simulink library "SMC"  (R2017b)
settings: Solver=VariableStepAuto  StartTime=0.0  StopTime=10.0  RelTol=1e-3
undefined symbols (not defined in the file or in its folder): A, B, beta, C, C0, filter, gamma0, K0, k02, K1, K2, K3, p, P2, PC, Pk, pk, rho, S, Slat, yc
libraries: dspmtrx3 x18
settings Model: Creator=lev201  LastModifiedBy=Liam Uni

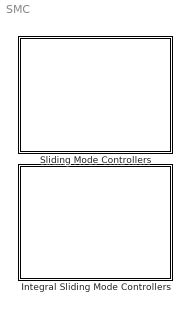
== system SMC ==
  Integral Sliding Mode Controllers : Subsystem
      mask Display: disp('Integral Sliding Mode Controllers')
  Sliding Mode Controllers : Subsystem
      mask Display: disp('Sliding Mode Controllers')

== system SMC/Integral Sliding Mode Controllers ==
  AISMC : Subsystem  mask{A=A, B=B, C=C, S=S, rho=rho, P2=P2, delta=0, eps=0, c0=C0, k0=K0, pc=PC, pk=Pk, filter=filter, yc=0}
      mask prompts: A "System Matrix (A)"; B "Effectiveness Matrix (B)"; C "Output Matrix (C)"; S "Sliding Surface (S)"; pc "Learning rate of c estimate"; pk "Learning rate of k estimation"
      mask init:
      | [K1 K2 K3]=SMCgains(S, A, B, C, yc, P2)
      mask DialogControl DescGroupVar Prompt: Adaptive Integral Sliding Mode Controller
      mask DialogControl DescTextVar Prompt: This controller gaurantees sliding as long as: rho>=||uncertainty|| A sigmoidal function can be used to create a continuous pseudo-sliding non-linear component using delta: sig(s)=P2s/(||P2s||+delta). A boundary layer around the sliding surface can be used using eps: if ||P2s||>eps un(t)=un(t) if ||P2s||<=eps, un(t)=0. An adaptive method is used to estimate the bounds of matched uncertaintym such that ||fm(x,u,t)||<=C1+K1||x(t)||. Integral action is introduced for the outputs yc.
      mask DialogControl Container4 Prompt: Model Parameters
      mask DialogControl Container6 Prompt: Controller Parameters
      mask DialogControl Container11 Prompt: Gain Tuning
      mask DialogControl Container12 Prompt: Chattering Avoidance
      mask DialogControl Container14 Prompt: Adaptive Parmeters
      mask DialogControl Container15 Prompt: Reference Tracking
      mask Display:
      | disp('AISMC')
      | port_label('input', 1, 'x(t)');
      | port_label('output', 1, 'u(t)');
      | port_label('output', 2, 's(t)');
      | port_label('output', 3, 'AP');
      | port_label('input', 2, 'R(t)');
  ISMC : Subsystem  mask{A=A, B=B, C=C, S=S, rho=rho, P2=P2, delta=0, eps=0, filter=filter, yc=yc}
      mask prompts: A "System Matrix (A)"; B "Effectiveness Matrix (B)"; C "Output Matrix (C)"; S "Sliding Surface (S)"
      mask init:
      | [K1 K2 K3]=SMCgains(S, A, B, C, yc, P2)
      mask DialogControl DescGroupVar Prompt: Integral Sliding Mode Controller
      mask DialogControl DescTextVar Prompt: This controller gaurantees sliding as long as: rho>=||uncertainty|| A sigmoidal function can be used to create a continuous pseudo-sliding non-linear component using delta: sig(s)=P2s/(||P2s||+delta).  A boundary layer around the sliding surface can be used using eps: if ||P2s||>eps un(t)=un(t) if ||P2s||<=eps un(t)=0. Integral action is introduced for the outputs yc.
      mask DialogControl Container4 Prompt: Model Parameters
      mask DialogControl Container6 Prompt: Controller Parameters
      mask DialogControl Container11 Prompt: Gain Tuning
      mask DialogControl Container12 Prompt: Chattering Avoidance
      mask DialogControl Container13 Prompt: Reference Tracking
      mask Display:
      | disp('ISMC')
      | port_label('input', 1, 'x(t)');
      | port_label('input', 2, 'R(t)');
      | 
      | port_label('output', 1, 'u(t)');
      | port_label('output', 2, 's(t)');
  SRAISMC : Subsystem  mask{A=A, B=B, C=C, S=S, rho=rho, P2=P2, delta=0, eps=0, c0=C0, gamma0=gamma0, pc=PC, beta=beta, filter=filter, yc=yc}
      mask prompts: A "System Matrix (A)"; B "Effectiveness Matrix (B)"; C "Output  Matrix (C)"; S "Sliding Surface (S)"; pc "Learning rate of c estimate"; beta "Adaptive rate"
      mask init:
      | [K1 K2 K3]=SMCgains(S, A, B, C, yc, P2)
      mask DialogControl DescGroupVar Prompt: Saturation Robust Adaptive Integral Sliding Mode Controller
      mask DialogControl DescTextVar Prompt: This controller gaurantees sliding as long as: rho>=||uncertainty|| A sigmoidal function can be used to create a continuous pseudo-sliding non-linear component using delta: sig(s)=P2s/(||P2s||+delta). A boundary layer around the sliding surface can be used using eps: if ||P2s||>eps un(t)=un(t) if ||P2s||<=eps, un(t)=0. An adaptive method is used to estimate the bounds of matched uncertaintym such that ||fm(x,u,t)||<=C1+K1||x(t)||.
      mask DialogControl Container4 Prompt: Model Parameters
      mask DialogControl Container6 Prompt: Controller Parameters
      mask DialogControl Container11 Prompt: Gain Tuning
      mask DialogControl Container12 Prompt: Chattering Avoidance
      mask DialogControl Container14 Prompt: Adaptive Parmeters
      mask DialogControl Container15 Prompt: Reference Tracking
      mask Display:
      | disp('SRAISMC')
      | port_label('input', 1, 'x(t)');
      | port_label('output', 1, 'u(t)');
      | port_label('output', 2, 's(t)');
      | port_label('output', 3, 'AP');
      | port_label('input', 2, 'R(t)');

== system SMC/Sliding Mode Controllers ==
  ASMC : Subsystem  mask{A=A, B=B, S=S, rho=rho, P2=P2, delta=0, eps=0, c0=C0, k0=K0, pc=PC, pk=Pk}
      mask prompts: A "System Matrix (A)"; B "Effectiveness Matrix (B)"; S "Sliding Surface (S)"; pc "Learning rate of c estimate"; pk "Learning rate of k estimation"
      mask init:
      | [K1 K2]=SMCgains(S, A, B, P2)
      mask DialogControl DescGroupVar Prompt: Adaptive Sliding Mode Controller
      mask DialogControl DescTextVar Prompt: This controller gaurantees sliding as long as: rho>=||uncertainty|| A sigmoidal function can be used to create a continuous pseudo-sliding non-linear component using delta: sig(s)=P2s/(||P2s||+delta). A boundary layer around the sliding surface can be used using eps: if ||P2s||>eps un(t)=un(t) if ||P2s||<=eps, un(t)=0. An adaptive method is used to estimate the bounds of matched uncertaintym such that ||fm(x,u,t)||<=C1+K1||x(t)||.
      mask DialogControl Container4 Prompt: Model Parameters
      mask DialogControl Container6 Prompt: Controller Parameters
      mask DialogControl Container11 Prompt: Gain Tuning
      mask DialogControl Container12 Prompt: Chattering Avoidance
      mask DialogControl Container14 Prompt: Adaptive Parmeters
      mask Display:
      | disp('ASMC')
      | port_label('input', 1, 'x(t)');
      | port_label('output', 1, 'u(t)');
      | port_label('output', 2, 's(t)');
      | port_label('output', 3, 'AP');
  SMC : Subsystem  mask{A=A, B=B, S=S, rho=rho, P2=P2, delta=0, eps=0}
      mask prompts: A "System Matrix (A)"; B "Effectiveness Matrix (B)"; S "Sliding Surface (S)"
      mask init:
      | [K1 K2]=SMCgains(S, A, B, P2)
      mask DialogControl DescGroupVar Prompt: Sliding Mode Controller
      mask DialogControl DescTextVar Prompt: This controller gaurantees sliding as long as: rho>=||uncertainty|| A sigmoidal function can be used to create a continuous pseudo-sliding non-linear component using delta: sig(s)=P2s/(||P2s||+delta).  A boundary layer around the sliding surface can be used using eps: if ||P2s||>eps un(t)=un(t) if ||P2s||<=eps un(t)=0
      mask DialogControl Container4 Prompt: Model Parameters
      mask DialogControl Container6 Prompt: Controller Parameters
      mask DialogControl Container11 Prompt: Gain Tuning
      mask DialogControl Container12 Prompt: Chattering Avoidance
      mask Display:
      | disp('SMC')
      | port_label('input', 1, 'x(t)');
      | port_label('output', 1, 'u(t)');
      | port_label('output', 2, 's(t)');
  SRASMC : Subsystem  mask{A=A, B=B, S=S, rho=rho, P2=P2, delta=0, eps=0, c0=C0, gamma0=gamma0, pc=PC, beta=beta}
      mask prompts: A "System Matrix (A)"; B "Effectiveness Matrix (B)"; S "Sliding Surface (S)"; pc "Learning rate of c estimate"; beta "Adaptive rate"
      mask init:
      | [K1 K2]=SMCgains(S, A, B, P2)
      mask DialogControl DescGroupVar Prompt: Saturation Robust Adaptive Sliding Mode Controller
      mask DialogControl DescTextVar Prompt: This controller gaurantees sliding as long as: rho>=||uncertainty|| A sigmoidal function can be used to create a continuous pseudo-sliding non-linear component using delta: sig(s)=P2s/(||P2s||+delta). A boundary layer around the sliding surface can be used using eps: if ||P2s||>eps un(t)=un(t) if ||P2s||<=eps, un(t)=0. An adaptive method is used to estimate the bounds of matched uncertaintym such that ||fm(x,u,t)||<=C1+K1||x(t)||.
      mask DialogControl Container4 Prompt: Model Parameters
      mask DialogControl Container6 Prompt: Controller Parameters
      mask DialogControl Container11 Prompt: Gain Tuning
      mask DialogControl Container12 Prompt: Chattering Avoidance
      mask DialogControl Container14 Prompt: Adaptive Parmeters
      mask Display:
      | disp('SRASMC')
      | port_label('input', 1, 'x(t)');
      | port_label('output', 1, 'u(t)');
      | port_label('output', 2, 's(t)');
      | port_label('output', 3, 'AP');

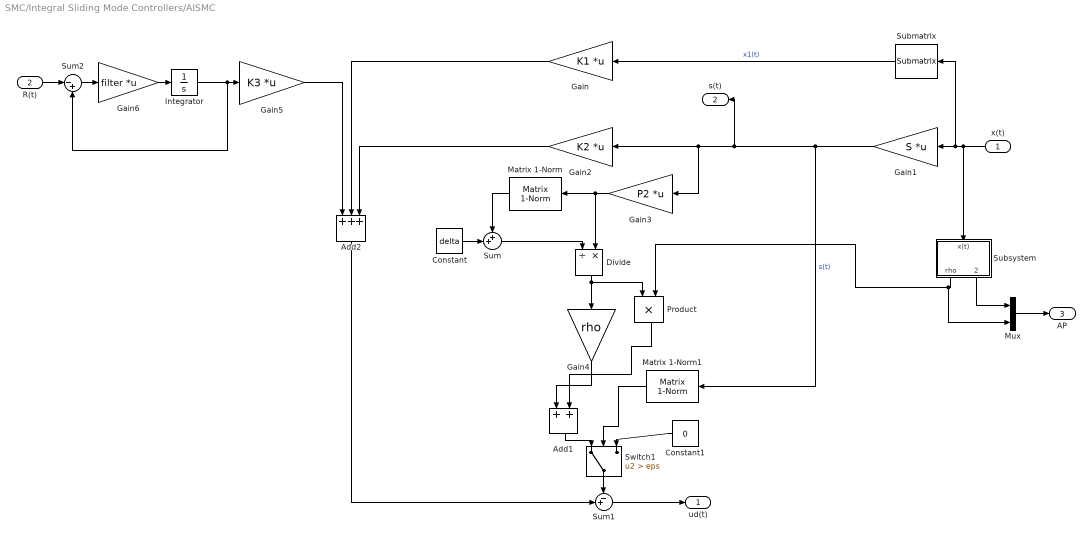
== system SMC/Integral Sliding Mode Controllers/AISMC ==
  x(t) : Inport
  R(t) : Inport  Port=2
  Add1 : Sum
  Add2 : Sum  Inputs=+++
  Constant : Constant  Value=delta
  Constant1 : Constant  Value=0
  Divide : Product  Inputs=/*
  Gain : Gain  Gain=K1  Multiplication=Matrix(K*u) (u vector)
  Gain1 : Gain  Gain=S  Multiplication=Matrix(K*u) (u vector)
  Gain2 : Gain  Gain=K2  Multiplication=Matrix(K*u) (u vector)
  Gain3 : Gain  Gain=P2  Multiplication=Matrix(K*u) (u vector)
  Gain4 : Gain  Gain=rho
  Gain5 : Gain  Gain=K3  Multiplication=Matrix(K*u) (u vector)
  Gain6 : Gain  Gain=filter  Multiplication=Matrix(K*u) (u vector)
  Integrator : Integrator
  Matrix 1-Norm : dspmtrx3/Matrix  1-Norm  outputDataTypeStr=Inherit: Same as accumulator  outputLastDataTypeStr=Inherit: Same as accumulator  outputMin=[]  outputMax=[]  roundingMode=Floor  overflowMode=off
      settings: SourceProductName=DSP System Toolbox  SourceProductBaseCode=DS
  Matrix 1-Norm1 : dspmtrx3/Matrix  1-Norm  outputDataTypeStr=Inherit: Same as accumulator  outputLastDataTypeStr=Inherit: Same as accumulator  outputMin=[]  outputMax=[]  roundingMode=Floor  overflowMode=off
      settings: SourceProductName=DSP System Toolbox  SourceProductBaseCode=DS
  Mux : Mux  Inputs=2
  Product : Product
  Submatrix : dspmtrx3/Submatrix  RowSpan=Range of rows  RowStartMode=Index  RowStartIndex=1  RowEndMode=Index  RowEndIndex=p-1  ColSpan=All columns  ColStartMode=First  ColStartIndex=1  ColEndMode=Last  ColEndIndex=1
  Subsystem : Subsystem
  Sum : Sum  Inputs=++|
  Sum1 : Sum  Inputs=-+|
  Sum2 : Sum  Inputs=|-+
  Switch1 : Switch  Criteria=u2 > Threshold  Threshold=eps  ZeroCross=off
  ud(t) : Outport
  s(t) : Outport  Port=2
  AP : Outport  Port=3
  wires:
  Gain1/1 -> Matrix 1-Norm1/1, Gain2/1, Gain3/1, s(t)/1  "s(t)"
  Divide/1 -> Product/1, Gain4/1
  Constant/1 -> Sum/2
  Matrix 1-Norm/1 -> Sum/1
  Gain4/1 -> Add1/1
  Sum/1 -> Divide/1
  Sum1/1 -> ud(t)/1
  Gain3/1 -> Matrix 1-Norm/1, Divide/2
  Switch1/1 -> Sum1/1
  Matrix 1-Norm1/1 -> Switch1/2
  Constant1/1 -> Switch1/3
  x(t)/1 -> Subsystem/1(x(t)), Submatrix/1, Gain1/1
  Submatrix/1 -> Gain/1  "x1(t)"
  Subsystem/1(rho) -> Mux/2, Product/2
  Add1/1 -> Switch1/1
  Product/1 -> Add1/2
  Subsystem/2(est-par) -> Mux/1
  Mux/1 -> AP/1
  Sum2/1 -> Gain6/1
  Gain5/1 -> Add2/1
  Gain6/1 -> Integrator/1
  Add2/1 -> Sum1/2
  Gain2/1 -> Add2/3
  Gain/1 -> Add2/2
  Integrator/1 -> Sum2/2, Gain5/1
  R(t)/1 -> Sum2/1

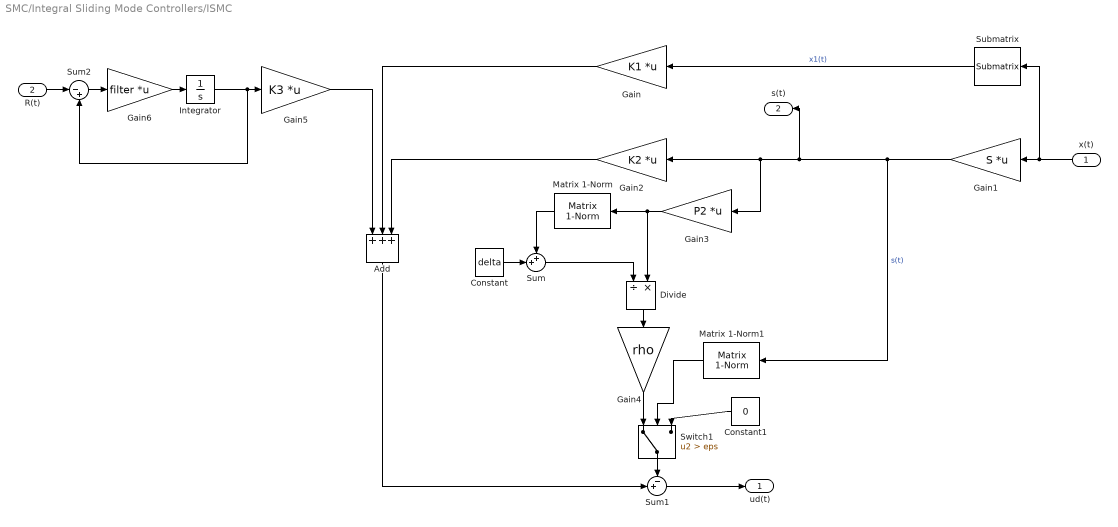
== system SMC/Integral Sliding Mode Controllers/ISMC ==
  x(t) : Inport
  R(t) : Inport  Port=2
  Add : Sum  Inputs=+++
  Constant : Constant  Value=delta
  Constant1 : Constant  Value=0
  Divide : Product  Inputs=/*
  Gain : Gain  Gain=K1  Multiplication=Matrix(K*u) (u vector)
  Gain1 : Gain  Gain=S  Multiplication=Matrix(K*u) (u vector)
  Gain2 : Gain  Gain=K2  Multiplication=Matrix(K*u) (u vector)
  Gain3 : Gain  Gain=P2  Multiplication=Matrix(K*u) (u vector)
  Gain4 : Gain  Gain=rho
  Gain5 : Gain  Gain=K3  Multiplication=Matrix(K*u) (u vector)
  Gain6 : Gain  Gain=filter  Multiplication=Matrix(K*u) (u vector)
  Integrator : Integrator
  Matrix 1-Norm : dspmtrx3/Matrix  1-Norm  outputDataTypeStr=Inherit: Same as accumulator  outputLastDataTypeStr=Inherit: Same as accumulator  outputMin=[]  outputMax=[]  roundingMode=Floor  overflowMode=off
      settings: SourceProductName=DSP System Toolbox  SourceProductBaseCode=DS
  Matrix 1-Norm1 : dspmtrx3/Matrix  1-Norm  outputDataTypeStr=Inherit: Same as accumulator  outputLastDataTypeStr=Inherit: Same as accumulator  outputMin=[]  outputMax=[]  roundingMode=Floor  overflowMode=off
      settings: SourceProductName=DSP System Toolbox  SourceProductBaseCode=DS
  Submatrix : dspmtrx3/Submatrix  RowSpan=Range of rows  RowStartMode=Index  RowStartIndex=1  RowEndMode=Index  RowEndIndex=p-1  ColSpan=All columns  ColStartMode=First  ColStartIndex=1  ColEndMode=Last  ColEndIndex=1
  Sum : Sum  Inputs=++|
  Sum1 : Sum  Inputs=-+|
  Sum2 : Sum  Inputs=|-+
  Switch1 : Switch  Criteria=u2 > Threshold  Threshold=eps  ZeroCross=off
  ud(t) : Outport
  s(t) : Outport  Port=2
  wires:
  Gain1/1 -> Matrix 1-Norm1/1, Gain2/1, Gain3/1, s(t)/1  "s(t)"
  Divide/1 -> Gain4/1
  Constant/1 -> Sum/2
  Matrix 1-Norm/1 -> Sum/1
  Add/1 -> Sum1/2
  Gain2/1 -> Add/3
  Gain4/1 -> Switch1/1
  Sum/1 -> Divide/1
  Sum1/1 -> ud(t)/1
  Gain3/1 -> Matrix 1-Norm/1, Divide/2
  Switch1/1 -> Sum1/1
  Matrix 1-Norm1/1 -> Switch1/2
  Constant1/1 -> Switch1/3
  x(t)/1 -> Submatrix/1, Gain1/1
  Submatrix/1 -> Gain/1  "x1(t)"
  Gain/1 -> Add/2
  Integrator/1 -> Sum2/2, Gain5/1
  Gain5/1 -> Add/1
  R(t)/1 -> Sum2/1
  Sum2/1 -> Gain6/1
  Gain6/1 -> Integrator/1

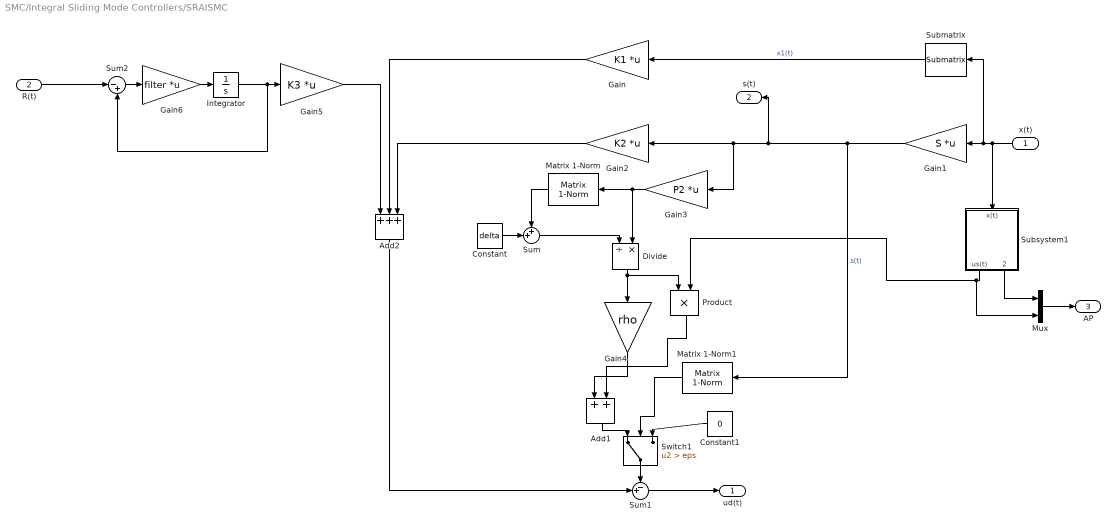
== system SMC/Integral Sliding Mode Controllers/SRAISMC ==
  x(t) : Inport
  R(t) : Inport  Port=2
  Add1 : Sum
  Add2 : Sum  Inputs=+++
  Constant : Constant  Value=delta
  Constant1 : Constant  Value=0
  Divide : Product  Inputs=/*
  Gain : Gain  Gain=K1  Multiplication=Matrix(K*u) (u vector)
  Gain1 : Gain  Gain=S  Multiplication=Matrix(K*u) (u vector)
  Gain2 : Gain  Gain=K2  Multiplication=Matrix(K*u) (u vector)
  Gain3 : Gain  Gain=P2  Multiplication=Matrix(K*u) (u vector)
  Gain4 : Gain  Gain=rho
  Gain5 : Gain  Gain=K3  Multiplication=Matrix(K*u) (u vector)
  Gain6 : Gain  Gain=filter  Multiplication=Matrix(K*u) (u vector)
  Integrator : Integrator
  Matrix 1-Norm : dspmtrx3/Matrix  1-Norm  outputDataTypeStr=Inherit: Same as accumulator  outputLastDataTypeStr=Inherit: Same as accumulator  outputMin=[]  outputMax=[]  roundingMode=Floor  overflowMode=off
      settings: SourceProductName=DSP System Toolbox  SourceProductBaseCode=DS
  Matrix 1-Norm1 : dspmtrx3/Matrix  1-Norm  outputDataTypeStr=Inherit: Same as accumulator  outputLastDataTypeStr=Inherit: Same as accumulator  outputMin=[]  outputMax=[]  roundingMode=Floor  overflowMode=off
      settings: SourceProductName=DSP System Toolbox  SourceProductBaseCode=DS
  Mux : Mux  Inputs=2
  Product : Product
  Submatrix : dspmtrx3/Submatrix  RowSpan=Range of rows  RowStartMode=Index  RowStartIndex=1  RowEndMode=Index  RowEndIndex=p-1  ColSpan=All columns  ColStartMode=First  ColStartIndex=1  ColEndMode=Last  ColEndIndex=1
  Subsystem1 : Subsystem
  Sum : Sum  Inputs=++|
  Sum1 : Sum  Inputs=-+|
  Sum2 : Sum  Inputs=|-+
  Switch1 : Switch  Criteria=u2 > Threshold  Threshold=eps  ZeroCross=off
  ud(t) : Outport
  s(t) : Outport  Port=2
  AP : Outport  Port=3
  wires:
  Mux/1 -> AP/1
  Subsystem1/2(est-par) -> Mux/1
  Product/1 -> Add1/2
  Add1/1 -> Switch1/1
  Subsystem1/1(us(t)) -> Product/2, Mux/2
  Gain/1 -> Add2/2
  Submatrix/1 -> Gain/1  "x1(t)"
  x(t)/1 -> Subsystem1/1(x(t)), Gain1/1, Submatrix/1
  Constant1/1 -> Switch1/3
  Matrix 1-Norm1/1 -> Switch1/2
  Switch1/1 -> Sum1/1
  Gain3/1 -> Divide/2, Matrix 1-Norm/1
  Sum1/1 -> ud(t)/1
  Sum/1 -> Divide/1
  Gain4/1 -> Add1/1
  Gain2/1 -> Add2/3
  Matrix 1-Norm/1 -> Sum/1
  Constant/1 -> Sum/2
  Divide/1 -> Gain4/1, Product/1
  Gain1/1 -> s(t)/1, Gain3/1, Gain2/1, Matrix 1-Norm1/1  "s(t)"
  Integrator/1 -> Sum2/2, Gain5/1
  R(t)/1 -> Sum2/1
  Gain6/1 -> Integrator/1
  Sum2/1 -> Gain6/1
  Gain5/1 -> Add2/1
  Add2/1 -> Sum1/2

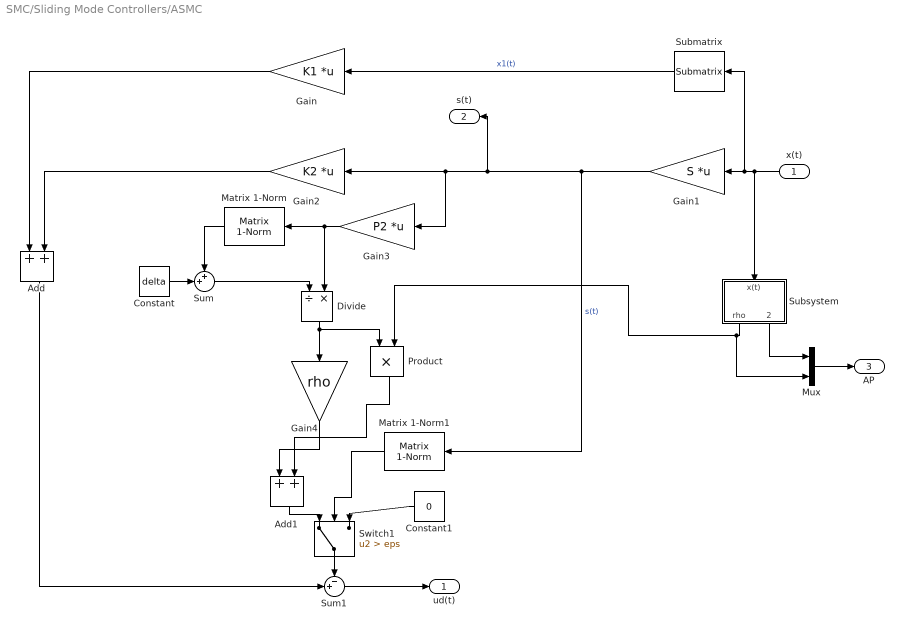
== system SMC/Sliding Mode Controllers/ASMC ==
  x(t) : Inport
  Add : Sum
  Add1 : Sum
  Constant : Constant  Value=delta
  Constant1 : Constant  Value=0
  Divide : Product  Inputs=/*
  Gain : Gain  Gain=K1  Multiplication=Matrix(K*u) (u vector)
  Gain1 : Gain  Gain=S  Multiplication=Matrix(K*u) (u vector)
  Gain2 : Gain  Gain=K2  Multiplication=Matrix(K*u) (u vector)
  Gain3 : Gain  Gain=P2  Multiplication=Matrix(K*u) (u vector)
  Gain4 : Gain  Gain=rho
  Matrix 1-Norm : dspmtrx3/Matrix  1-Norm  outputDataTypeStr=Inherit: Same as accumulator  outputLastDataTypeStr=Inherit: Same as accumulator  outputMin=[]  outputMax=[]  roundingMode=Floor  overflowMode=off
      settings: SourceProductName=DSP System Toolbox  SourceProductBaseCode=DS
  Matrix 1-Norm1 : dspmtrx3/Matrix  1-Norm  outputDataTypeStr=Inherit: Same as accumulator  outputLastDataTypeStr=Inherit: Same as accumulator  outputMin=[]  outputMax=[]  roundingMode=Floor  overflowMode=off
      settings: SourceProductName=DSP System Toolbox  SourceProductBaseCode=DS
  Mux : Mux  Inputs=2
  Product : Product
  Submatrix : dspmtrx3/Submatrix  RowSpan=Range of rows  RowStartMode=Index  RowStartIndex=1  RowEndMode=Index  RowEndIndex=p-1  ColSpan=All columns  ColStartMode=First  ColStartIndex=1  ColEndMode=Last  ColEndIndex=1
  Subsystem : Subsystem
  Sum : Sum  Inputs=++|
  Sum1 : Sum  Inputs=-+|
  Switch1 : Switch  Criteria=u2 > Threshold  Threshold=eps  ZeroCross=off
  ud(t) : Outport
  s(t) : Outport  Port=2
  AP : Outport  Port=3
  wires:
  Gain1/1 -> Matrix 1-Norm1/1, Gain2/1, Gain3/1, s(t)/1  "s(t)"
  Divide/1 -> Product/1, Gain4/1
  Constant/1 -> Sum/2
  Matrix 1-Norm/1 -> Sum/1
  Add/1 -> Sum1/2
  Gain2/1 -> Add/2
  Gain4/1 -> Add1/1
  Sum/1 -> Divide/1
  Sum1/1 -> ud(t)/1
  Gain3/1 -> Matrix 1-Norm/1, Divide/2
  Switch1/1 -> Sum1/1
  Matrix 1-Norm1/1 -> Switch1/2
  Constant1/1 -> Switch1/3
  x(t)/1 -> Subsystem/1(x(t)), Submatrix/1, Gain1/1
  Submatrix/1 -> Gain/1  "x1(t)"
  Gain/1 -> Add/1
  Subsystem/1(rho) -> Mux/2, Product/2
  Add1/1 -> Switch1/1
  Product/1 -> Add1/2
  Subsystem/2(est-par) -> Mux/1
  Mux/1 -> AP/1

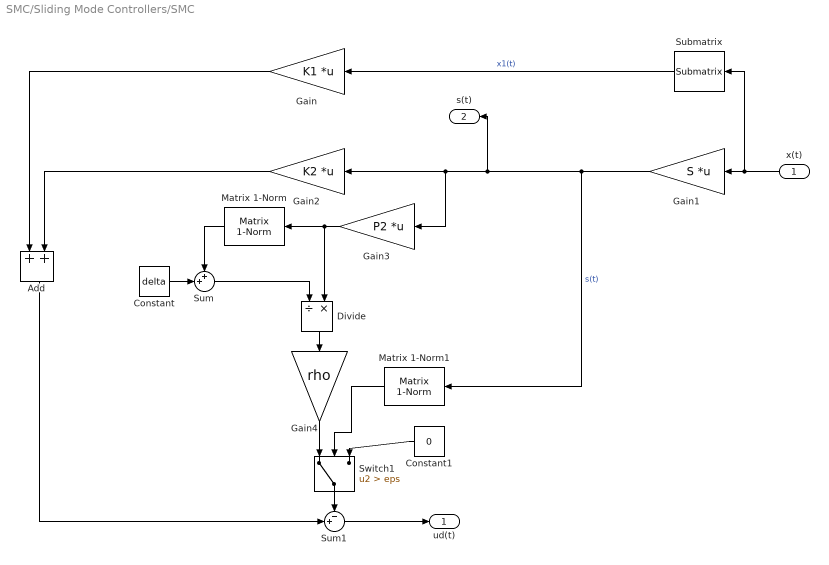
== system SMC/Sliding Mode Controllers/SMC ==
  x(t) : Inport
  Add : Sum
  Constant : Constant  Value=delta
  Constant1 : Constant  Value=0
  Divide : Product  Inputs=/*
  Gain : Gain  Gain=K1  Multiplication=Matrix(K*u) (u vector)
  Gain1 : Gain  Gain=S  Multiplication=Matrix(K*u) (u vector)
  Gain2 : Gain  Gain=K2  Multiplication=Matrix(K*u) (u vector)
  Gain3 : Gain  Gain=P2  Multiplication=Matrix(K*u) (u vector)
  Gain4 : Gain  Gain=rho
  Matrix 1-Norm : dspmtrx3/Matrix  1-Norm  outputDataTypeStr=Inherit: Same as accumulator  outputLastDataTypeStr=Inherit: Same as accumulator  outputMin=[]  outputMax=[]  roundingMode=Floor  overflowMode=off
      settings: SourceProductName=DSP System Toolbox  SourceProductBaseCode=DS
  Matrix 1-Norm1 : dspmtrx3/Matrix  1-Norm  outputDataTypeStr=Inherit: Same as accumulator  outputLastDataTypeStr=Inherit: Same as accumulator  outputMin=[]  outputMax=[]  roundingMode=Floor  overflowMode=off
      settings: SourceProductName=DSP System Toolbox  SourceProductBaseCode=DS
  Submatrix : dspmtrx3/Submatrix  RowSpan=Range of rows  RowStartMode=Index  RowStartIndex=1  RowEndMode=Index  RowEndIndex=p-1  ColSpan=All columns  ColStartMode=First  ColStartIndex=1  ColEndMode=Last  ColEndIndex=1
  Sum : Sum  Inputs=++|
  Sum1 : Sum  Inputs=-+|
  Switch1 : Switch  Criteria=u2 > Threshold  Threshold=eps  ZeroCross=off
  ud(t) : Outport
  s(t) : Outport  Port=2
  wires:
  Gain1/1 -> Matrix 1-Norm1/1, Gain2/1, Gain3/1, s(t)/1  "s(t)"
  Divide/1 -> Gain4/1
  Constant/1 -> Sum/2
  Matrix 1-Norm/1 -> Sum/1
  Add/1 -> Sum1/2
  Gain2/1 -> Add/2
  Gain4/1 -> Switch1/1
  Sum/1 -> Divide/1
  Sum1/1 -> ud(t)/1
  Gain3/1 -> Matrix 1-Norm/1, Divide/2
  Switch1/1 -> Sum1/1
  Matrix 1-Norm1/1 -> Switch1/2
  Constant1/1 -> Switch1/3
  x(t)/1 -> Submatrix/1, Gain1/1
  Submatrix/1 -> Gain/1  "x1(t)"
  Gain/1 -> Add/1

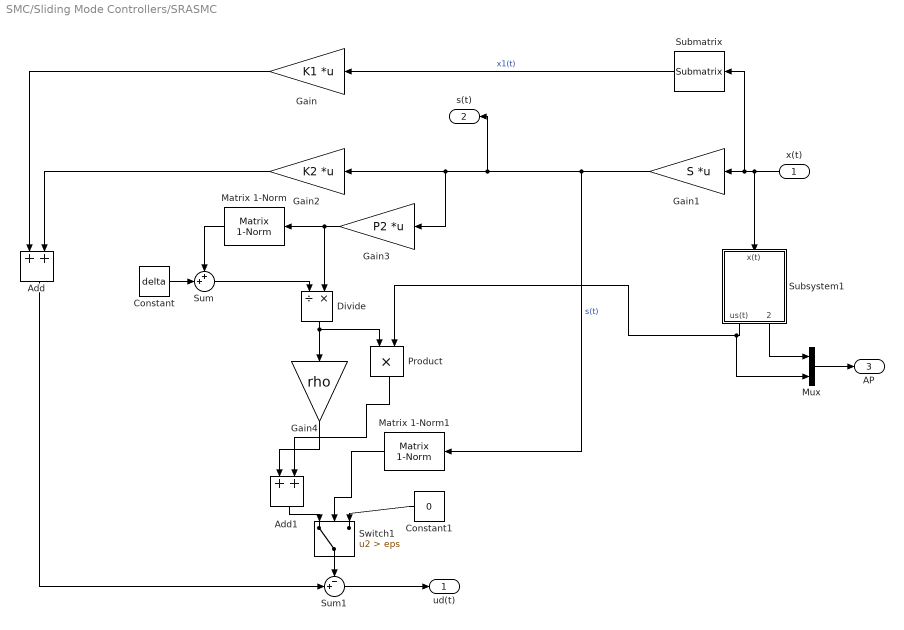
== system SMC/Sliding Mode Controllers/SRASMC ==
  x(t) : Inport
  Add : Sum
  Add1 : Sum
  Constant : Constant  Value=delta
  Constant1 : Constant  Value=0
  Divide : Product  Inputs=/*
  Gain : Gain  Gain=K1  Multiplication=Matrix(K*u) (u vector)
  Gain1 : Gain  Gain=S  Multiplication=Matrix(K*u) (u vector)
  Gain2 : Gain  Gain=K2  Multiplication=Matrix(K*u) (u vector)
  Gain3 : Gain  Gain=P2  Multiplication=Matrix(K*u) (u vector)
  Gain4 : Gain  Gain=rho
  Matrix 1-Norm : dspmtrx3/Matrix  1-Norm  outputDataTypeStr=Inherit: Same as accumulator  outputLastDataTypeStr=Inherit: Same as accumulator  outputMin=[]  outputMax=[]  roundingMode=Floor  overflowMode=off
      settings: SourceProductName=DSP System Toolbox  SourceProductBaseCode=DS
  Matrix 1-Norm1 : dspmtrx3/Matrix  1-Norm  outputDataTypeStr=Inherit: Same as accumulator  outputLastDataTypeStr=Inherit: Same as accumulator  outputMin=[]  outputMax=[]  roundingMode=Floor  overflowMode=off
      settings: SourceProductName=DSP System Toolbox  SourceProductBaseCode=DS
  Mux : Mux  Inputs=2
  Product : Product
  Submatrix : dspmtrx3/Submatrix  RowSpan=Range of rows  RowStartMode=Index  RowStartIndex=1  RowEndMode=Index  RowEndIndex=p-1  ColSpan=All columns  ColStartMode=First  ColStartIndex=1  ColEndMode=Last  ColEndIndex=1
  Subsystem1 : Subsystem
  Sum : Sum  Inputs=++|
  Sum1 : Sum  Inputs=-+|
  Switch1 : Switch  Criteria=u2 > Threshold  Threshold=eps  ZeroCross=off
  ud(t) : Outport
  s(t) : Outport  Port=2
  AP : Outport  Port=3
  wires:
  Mux/1 -> AP/1
  Subsystem1/2(est-par) -> Mux/1
  Product/1 -> Add1/2
  Add1/1 -> Switch1/1
  Subsystem1/1(us(t)) -> Product/2, Mux/2
  Gain/1 -> Add/1
  Submatrix/1 -> Gain/1  "x1(t)"
  x(t)/1 -> Subsystem1/1(x(t)), Gain1/1, Submatrix/1
  Constant1/1 -> Switch1/3
  Matrix 1-Norm1/1 -> Switch1/2
  Switch1/1 -> Sum1/1
  Gain3/1 -> Divide/2, Matrix 1-Norm/1
  Sum1/1 -> ud(t)/1
  Sum/1 -> Divide/1
  Gain4/1 -> Add1/1
  Gain2/1 -> Add/2
  Add/1 -> Sum1/2
  Matrix 1-Norm/1 -> Sum/1
  Constant/1 -> Sum/2
  Divide/1 -> Gain4/1, Product/1
  Gain1/1 -> s(t)/1, Gain3/1, Gain2/1, Matrix 1-Norm1/1  "s(t)"

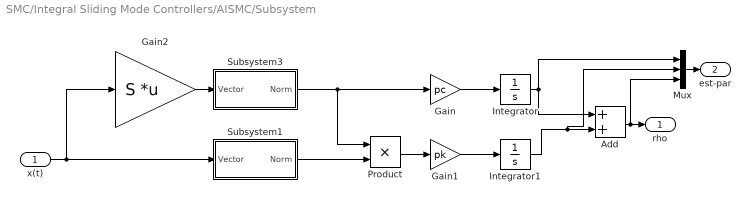
== system SMC/Integral Sliding Mode Controllers/AISMC/Subsystem ==
  x(t) : Inport
  Add : Sum
  Gain : Gain  Gain=pc
  Gain1 : Gain  Gain=pk
  Gain2 : Gain  Gain=S  Multiplication=Matrix(K*u) (u vector)
  Integrator : Integrator  InitialCondition=c0
  Integrator1 : Integrator  InitialCondition=k0
  Mux : Mux  Inputs=3
  Product : Product
  Subsystem1 : Subsystem
  Subsystem3 : Subsystem
  rho : Outport
  est-par : Outport  Port=2
  wires:
  Gain/1 -> Integrator/1
  Integrator/1 -> Add/1, Mux/1
  Subsystem3/1(Norm) -> Product/1, Gain/1
  x(t)/1 -> Subsystem1/1(Vector), Gain2/1
  Subsystem1/1(Norm) -> Product/2
  Product/1 -> Gain1/1
  Gain1/1 -> Integrator1/1
  Add/1 -> Mux/3, rho/1
  Integrator1/1 -> Mux/2, Add/2
  Gain2/1 -> Subsystem3/1(Vector)
  Mux/1 -> est-par/1

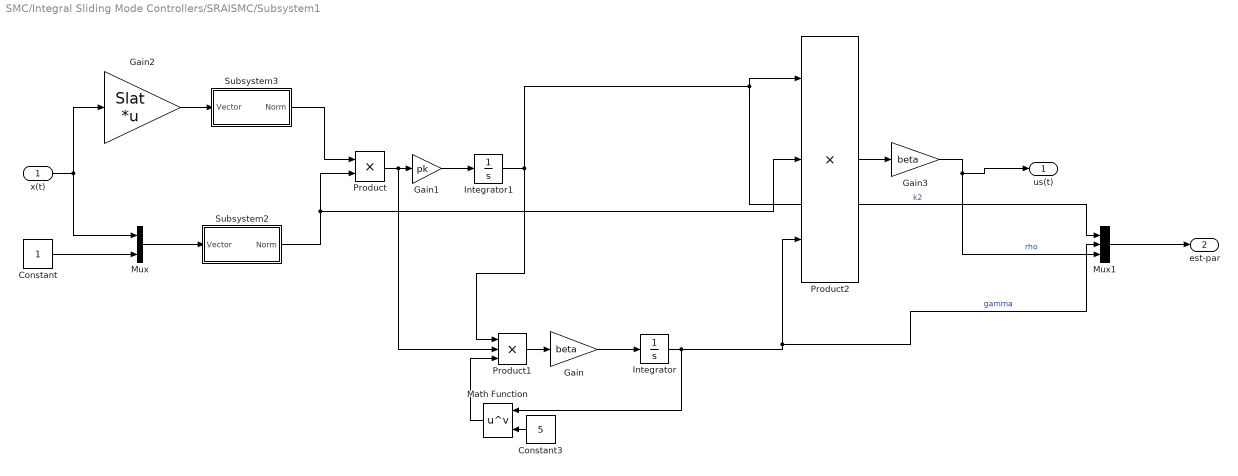
== system SMC/Integral Sliding Mode Controllers/SRAISMC/Subsystem1 ==
  x(t) : Inport
  Constant : Constant
  Constant3 : Constant  Value=5
  Gain : Gain  Gain=beta
  Gain1 : Gain  Gain=pk
  Gain2 : Gain  Gain=Slat  Multiplication=Matrix(K*u) (u vector)
  Gain3 : Gain  Gain=beta
  Integrator : Integrator  InitialCondition=gamma0
  Integrator1 : Integrator  InitialCondition=k02
  Math Function : Math  Operator=pow  SaturateOnIntegerOverflow=on
  Mux : Mux  Inputs=2
  Mux1 : Mux  Inputs=3
  Product : Product
  Product1 : Product  Inputs=3
  Product2 : Product  Inputs=3
  Subsystem2 : Subsystem
  Subsystem3 : Subsystem
  us(t) : Outport
  est-par : Outport  Port=2
  wires:
  Integrator/1 -> Mux1/2, Product2/3, Math Function/1  "gamma"
  Subsystem3/1(Norm) -> Product/1
  x(t)/1 -> Mux/1, Gain2/1
  Subsystem2/1(Norm) -> Product2/2, Product/2
  Product/1 -> Product1/2, Gain1/1
  Gain1/1 -> Integrator1/1
  Integrator1/1 -> Mux1/1, Product2/1, Product1/1  "k2"
  Gain2/1 -> Subsystem3/1(Vector)
  Mux/1 -> Subsystem2/1(Vector)
  Constant/1 -> Mux/2
  Product1/1 -> Gain/1
  Product2/1 -> Gain3/1
  Gain3/1 -> us(t)/1, Mux1/3  "rho"
  Gain/1 -> Integrator/1
  Constant3/1 -> Math Function/2
  Math Function/1 -> Product1/3
  Mux1/1 -> est-par/1

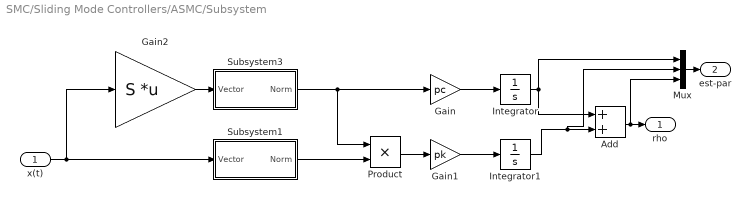
== system SMC/Sliding Mode Controllers/ASMC/Subsystem ==
  x(t) : Inport
  Add : Sum
  Gain : Gain  Gain=pc
  Gain1 : Gain  Gain=pk
  Gain2 : Gain  Gain=S  Multiplication=Matrix(K*u) (u vector)
  Integrator : Integrator  InitialCondition=c0
  Integrator1 : Integrator  InitialCondition=k0
  Mux : Mux  Inputs=3
  Product : Product
  Subsystem1 : Subsystem
  Subsystem3 : Subsystem
  rho : Outport
  est-par : Outport  Port=2
  wires:
  Gain/1 -> Integrator/1
  Integrator/1 -> Add/1, Mux/1
  Subsystem3/1(Norm) -> Product/1, Gain/1
  x(t)/1 -> Subsystem1/1(Vector), Gain2/1
  Subsystem1/1(Norm) -> Product/2
  Product/1 -> Gain1/1
  Gain1/1 -> Integrator1/1
  Add/1 -> Mux/3, rho/1
  Integrator1/1 -> Mux/2, Add/2
  Gain2/1 -> Subsystem3/1(Vector)
  Mux/1 -> est-par/1

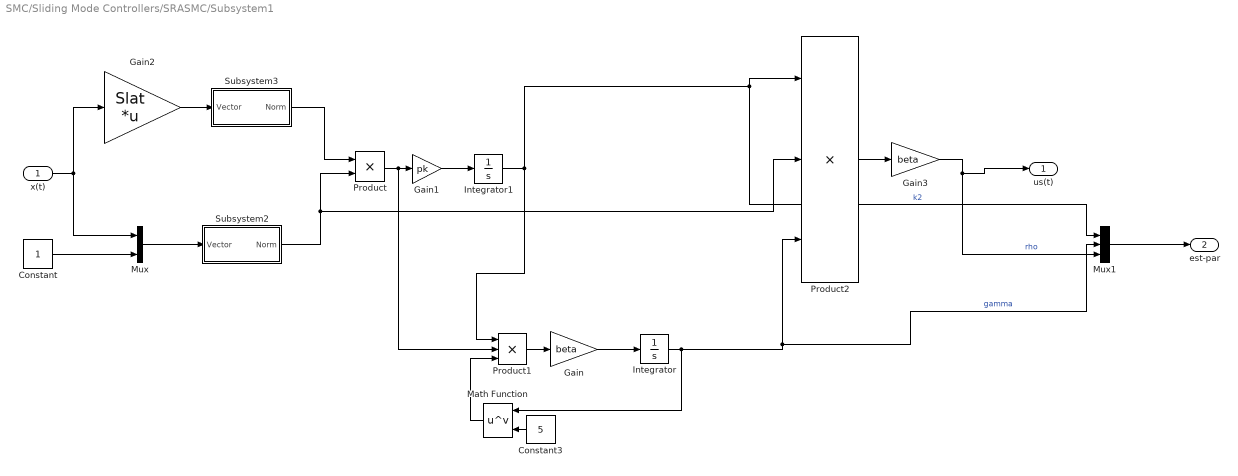
== system SMC/Sliding Mode Controllers/SRASMC/Subsystem1 ==
  x(t) : Inport
  Constant : Constant
  Constant3 : Constant  Value=5
  Gain : Gain  Gain=beta
  Gain1 : Gain  Gain=pk
  Gain2 : Gain  Gain=Slat  Multiplication=Matrix(K*u) (u vector)
  Gain3 : Gain  Gain=beta
  Integrator : Integrator  InitialCondition=gamma0
  Integrator1 : Integrator  InitialCondition=k02
  Math Function : Math  Operator=pow  SaturateOnIntegerOverflow=on
  Mux : Mux  Inputs=2
  Mux1 : Mux  Inputs=3
  Product : Product
  Product1 : Product  Inputs=3
  Product2 : Product  Inputs=3
  Subsystem2 : Subsystem
  Subsystem3 : Subsystem
  us(t) : Outport
  est-par : Outport  Port=2
  wires:
  Integrator/1 -> Mux1/2, Product2/3, Math Function/1  "gamma"
  Subsystem3/1(Norm) -> Product/1
  x(t)/1 -> Mux/1, Gain2/1
  Subsystem2/1(Norm) -> Product2/2, Product/2
  Product/1 -> Product1/2, Gain1/1
  Gain1/1 -> Integrator1/1
  Integrator1/1 -> Mux1/1, Product2/1, Product1/1  "k2"
  Gain2/1 -> Subsystem3/1(Vector)
  Mux/1 -> Subsystem2/1(Vector)
  Constant/1 -> Mux/2
  Product1/1 -> Gain/1
  Product2/1 -> Gain3/1
  Gain3/1 -> us(t)/1, Mux1/3  "rho"
  Gain/1 -> Integrator/1
  Constant3/1 -> Math Function/2
  Math Function/1 -> Product1/3
  Mux1/1 -> est-par/1

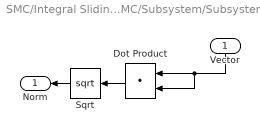
== system SMC/Integral Sliding Mode Controllers/AISMC/Subsystem/Subsystem1 ==
  Vector : Inport
  Dot Product : DotProduct  InputSameDT=on  OutDataTypeStr=Inherit: Inherit via internal rule
  Sqrt : Sqrt  SaturateOnIntegerOverflow=on
  Norm : Outport
  wires:
  Dot Product/1 -> Sqrt/1
  Sqrt/1 -> Norm/1
  Vector/1 -> Dot Product/2, Dot Product/1

== system SMC/Integral Sliding Mode Controllers/AISMC/Subsystem/Subsystem3 ==
  Vector : Inport
  Dot Product : DotProduct  InputSameDT=on  OutDataTypeStr=Inherit: Inherit via internal rule
  Sqrt : Sqrt  SaturateOnIntegerOverflow=on
  Norm : Outport
  wires:
  Dot Product/1 -> Sqrt/1
  Sqrt/1 -> Norm/1
  Vector/1 -> Dot Product/2, Dot Product/1

== system SMC/Integral Sliding Mode Controllers/SRAISMC/Subsystem1/Subsystem2 ==
  Vector : Inport
  Dot Product : DotProduct  InputSameDT=on  OutDataTypeStr=Inherit: Inherit via internal rule
  Sqrt : Sqrt  SaturateOnIntegerOverflow=on
  Norm : Outport
  wires:
  Dot Product/1 -> Sqrt/1
  Sqrt/1 -> Norm/1
  Vector/1 -> Dot Product/2, Dot Product/1

== system SMC/Integral Sliding Mode Controllers/SRAISMC/Subsystem1/Subsystem3 ==
  Vector : Inport
  Dot Product : DotProduct  InputSameDT=on  OutDataTypeStr=Inherit: Inherit via internal rule
  Sqrt : Sqrt  SaturateOnIntegerOverflow=on
  Norm : Outport
  wires:
  Dot Product/1 -> Sqrt/1
  Sqrt/1 -> Norm/1
  Vector/1 -> Dot Product/2, Dot Product/1

== system SMC/Sliding Mode Controllers/ASMC/Subsystem/Subsystem1 ==
  Vector : Inport
  Dot Product : DotProduct  InputSameDT=on  OutDataTypeStr=Inherit: Inherit via internal rule
  Sqrt : Sqrt  SaturateOnIntegerOverflow=on
  Norm : Outport
  wires:
  Dot Product/1 -> Sqrt/1
  Sqrt/1 -> Norm/1
  Vector/1 -> Dot Product/2, Dot Product/1

== system SMC/Sliding Mode Controllers/ASMC/Subsystem/Subsystem3 ==
  Vector : Inport
  Dot Product : DotProduct  InputSameDT=on  OutDataTypeStr=Inherit: Inherit via internal rule
  Sqrt : Sqrt  SaturateOnIntegerOverflow=on
  Norm : Outport
  wires:
  Dot Product/1 -> Sqrt/1
  Sqrt/1 -> Norm/1
  Vector/1 -> Dot Product/2, Dot Product/1

== system SMC/Sliding Mode Controllers/SRASMC/Subsystem1/Subsystem2 ==
  Vector : Inport
  Dot Product : DotProduct  InputSameDT=on  OutDataTypeStr=Inherit: Inherit via internal rule
  Sqrt : Sqrt  SaturateOnIntegerOverflow=on
  Norm : Outport
  wires:
  Dot Product/1 -> Sqrt/1
  Sqrt/1 -> Norm/1
  Vector/1 -> Dot Product/2, Dot Product/1

== system SMC/Sliding Mode Controllers/SRASMC/Subsystem1/Subsystem3 ==
  Vector : Inport
  Dot Product : DotProduct  InputSameDT=on  OutDataTypeStr=Inherit: Inherit via internal rule
  Sqrt : Sqrt  SaturateOnIntegerOverflow=on
  Norm : Outport
  wires:
  Dot Product/1 -> Sqrt/1
  Sqrt/1 -> Norm/1
  Vector/1 -> Dot Product/2, Dot Product/1
